simulink model "modeloPreditivo"  (R2018b)
settings: Solver=VariableStepAuto  StartTime=0.0  StopTime=1000  RelTol=1e-3
values from neighbouring files (symbols this model uses):
  A = [0 1 0 0 ... (first row only)    [dadosBallBeam.m]    (also in dadosTanqueQuatro.m = [-1/T1 0 A3/(A1*T3) 0; tanqueQuatroLinearizacao.m = double(subs(As,{h1,h2,h3,h4,v1,v2},{h10,h20,h30,h40,v10,v20})
  B = [0 0 0 1]'    [dadosBallBeam.m]    (also in dadosTanqueQuatro.m = [(y1*k1)/A1 0; tanqueQuatroLinearizacao.m = double(subs(Bs,{h1,h2,h3,h4,v1,v2},{h10,h20,h30,h40,v10,v20})
  C = [1 0 0 0]    [dadosBallBeam.m]    (also in dadosTanqueQuatro.m = [1 0 0 0; tanqueQuatroLinearizacao.m = [1 0 0 0)
  D = [0]    [dadosBallBeam.m]    (also in dadosTanqueQuatro.m = [0 0; tanqueQuatroLinearizacao.m = [0 0)
  h = 0.1    [MPC_sem_restricao.m]
  Kmpc = Kmpc(1:n_entradas,:)    [MPC_sem_restricao.m]    (also in dados_MPC_com_restricao.m; dados_MPC_com_restricao_estimador.m; dados_MPC_sem_restricao.m; dados_MPC_sem_restricao_estimador.m)
  Rl = Cp*Ap    [MPC_sem_restricao.m]    (also in dados_MPC_com_restricao.m; dados_MPC_com_restricao_estimador.m; dados_MPC_sem_restricao.m; dados_MPC_sem_restricao_estimador.m)
  Wr = [Wr; eye(n_entradas)]    [MPC_sem_restricao.m]    (also in dados_MPC_com_restricao.m; dados_MPC_com_restricao_estimador.m; dados_MPC_sem_restricao.m; dados_MPC_sem_restricao_estimador.m)
undefined symbols (not defined in the file or in its folder): DiscIntNeverNeededParam
libraries: simulink x1
settings Model: Creator=Caléo  LastModifiedBy=Caléo

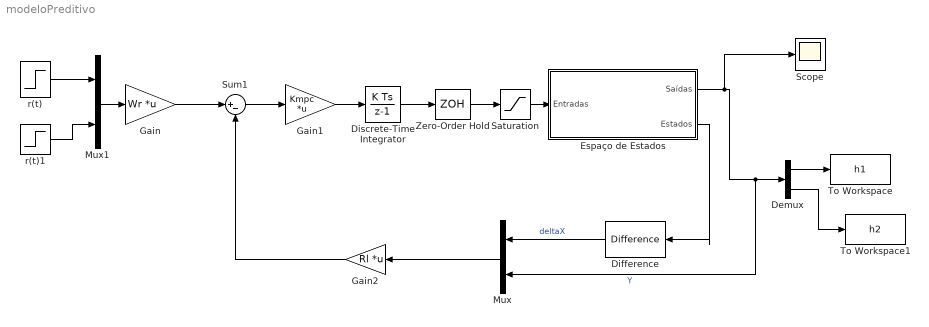
== system modeloPreditivo ==
  Demux : Demux  Outputs=2
  Difference : simulink/Discrete/Difference  ICPrevInput=0.0  OutMin=[]  OutMax=[]  OutDataType=fixdt(1, 16)  OutScaling=2^-10  DoSatur=off
  Discrete-Time Integrator : DiscreteIntegrator  SampleTime=h  ICPrevOutput=DiscIntNeverNeededParam  ICPrevScaledInput=DiscIntNeverNeededParam
  Espaço de Estados : Subsystem
  Gain : Gain  Gain=Wr  Multiplication=Matrix(K*u)
  Gain1 : Gain  Gain=Kmpc  Multiplication=Matrix(K*u)
  Gain2 : Gain  Gain=Rl  Multiplication=Matrix(K*u)
  Mux : Mux  Inputs=2
  Mux1 : Mux  Inputs=2
  Saturation : Saturate  UpperLimit=15  LowerLimit=-50
  Scope : Scope
  Sum1 : Sum  Inputs=|+-
  To Workspace : ToWorkspace  VariableName=h1  SaveFormat=Timeseries  SampleTime=-1
  To Workspace1 : ToWorkspace  VariableName=h2  SaveFormat=Timeseries  SampleTime=-1
  Zero-Order Hold : ZeroOrderHold  SampleTime=h
  r(t) : Step  Time=0  After=2  SampleTime=0
  r(t)1 : Step  Time=0  After=-0.5  SampleTime=0
  wires:
  Discrete-Time Integrator/1 -> Zero-Order Hold/1
  Espaço de Estados/1(Saídas) -> Scope/1, Mux/2, Demux/1  "Y"
  Difference/1 -> Mux/1  "deltaX"
  Demux/1 -> To Workspace/1
  Demux/2 -> To Workspace1/1
  Mux/1 -> Gain2/1
  Gain2/1 -> Sum1/2
  Gain1/1 -> Discrete-Time Integrator/1
  Sum1/1 -> Gain1/1
  Gain/1 -> Sum1/1
  Mux1/1 -> Gain/1
  r(t)/1 -> Mux1/1
  r(t)1/1 -> Mux1/2
  Zero-Order Hold/1 -> Saturation/1
  Saturation/1 -> Espaço de Estados/1(Entradas)
  Espaço de Estados/2(Estados) -> Difference/1

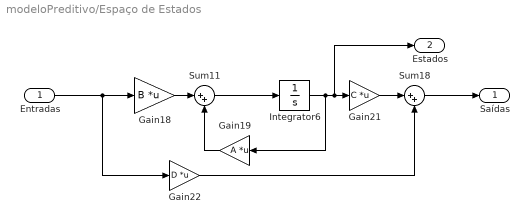
== system modeloPreditivo/Espaço de Estados ==
  Entradas : Inport
  Gain18 : Gain  Gain=B  Multiplication=Matrix(K*u)
  Gain19 : Gain  Gain=A  Multiplication=Matrix(K*u)
  Gain21 : Gain  Gain=C  Multiplication=Matrix(K*u)
  Gain22 : Gain  Gain=D  Multiplication=Matrix(K*u)
  Integrator6 : Integrator
  Sum11 : Sum  Inputs=|++
  Sum18 : Sum  Inputs=|++
  Saídas : Outport
  Estados : Outport  Port=2
  wires:
  Entradas/1 -> Gain22/1, Gain18/1
  Sum18/1 -> Saídas/1
  Gain22/1 -> Sum18/2
  Gain18/1 -> Sum11/1
  Gain19/1 -> Sum11/2
  Integrator6/1 -> Gain19/1, Estados/1, Gain21/1
  Sum11/1 -> Integrator6/1
  Gain21/1 -> Sum18/1
